simulink model "1SecondOrderUnderdampedSystem"  (R2023b)
settings: Solver=VariableStepAuto  StartTime=0.0  StopTime=10.0  RelTol=1e-3
undefined symbols (not defined in the file): G_den, G_num
settings Model: Creator=Patrick James  LastModifiedBy=Patrick James

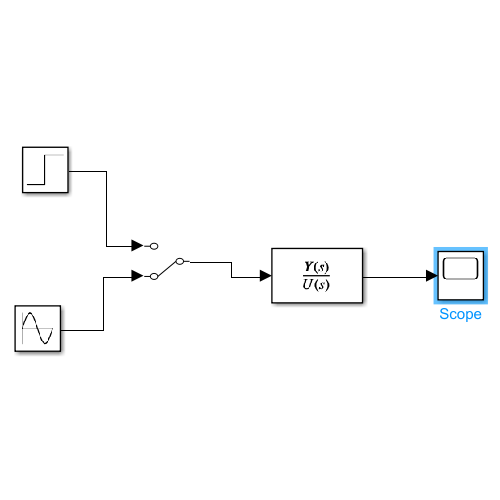
[thumbnail: Simulink's stored preview of the top-level diagram]
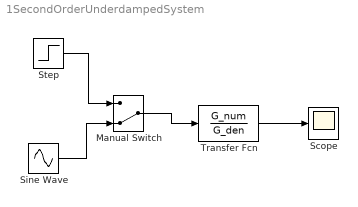
== system 1SecondOrderUnderdampedSystem ==
  Manual Switch : ManualSwitch  CurrentSetting=0
  Scope : Scope
  Sine Wave : Sin  SampleTime=0
  Step : Step  SampleTime=0
  Transfer Fcn : TransferFcn  Numerator=G_num  Denominator=G_den
  wires:
  Transfer Fcn/1 -> Scope/1
  Step/1 -> Manual Switch/1
  Sine Wave/1 -> Manual Switch/2
  Manual Switch/1 -> Transfer Fcn/1
